simulink model "CDPR_bloques_lazo_cerrado_R2020a"  (R2020b)
settings: Solver=ode15s  StartTime=0.0  StopTime=10  MaxStep=0.001  RelTol=1e-30
InitFcn:
  | % The global parameters for simulink are defined by running this script
  | % - Back emf constant           [Kb] (V/rad/sec)
  | % - Motor torque constant       [Kt] (N.m/A)
  | % - Mechanical inertia          [Jm] (kg.m^2)
  | % - Friction coeficient         [Bm] (N.m.s)
  | % - Armature resistance         [Ra] (Ohm)
  | % - Armature inductance         [La] (H)
  | 
  | Kb = 1.25;
  | Kt = 0.516;
  | Jm = 0.0221;
  | Bm = 0.002953;
  | Ra = 2.581;
  | La = 0.0281;
  | b = 0.1;
  | m = 0.5;
  | g = 9.81;
  | r = 0.3;
settings Model: OrderedModelArguments=off  Creator=C20256  LastModifiedBy=C20256
settings DebuggingCC: AlgebraicLoopMsg=none

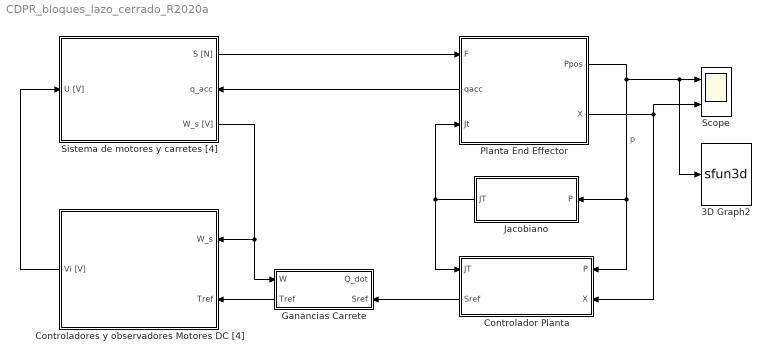
== system CDPR_bloques_lazo_cerrado_R2020a ==
  3D Graph2 : S-Function  LoadFcn=if exist('sfun3d','file'), sfun3d([],[],[],'LoadBlock'); end  FunctionName=sfun3d  Parameters=ax,T,np,cp,gd,ls,mk,mx,hd,tb  SFunctionDeploymentMode=off  EnableBusSupport=off  mask(3D Graph){np=1, ax=[-20 20 -20 20 0 20], mx=1e4, T=0.1, cp=[20 50 0.1], gd=on, hd=off, tb=off, ls=-, mk=none}
      mask prompts: np "Number of moving points (lines)"; ax "Range: [xmin xmax  ymin ymax zmin zmax]"; mx "Max number of points in each line"; T "Sampling Time"; cp "Camera position (use [0 0 1] for 2D XY view)"; gd "Grid (on|off)"; hd "HeadMarkers (on|off)"; tb "Toolbar (on|off)"; ls "LineStyle"; mk "LineMarker"
      mask help:
      | This block plots the position of several points in the XYZ space. The input contains the coordinates of all the points (x1,y1,z1,x2,y2,z2,...).
      | The number of moving points (lines), the XYZ ranges, sampling time, camera position, and grid (among other things) can be set as mask parameters.
      settings: CopyFcn=if exist('sfun3d','file'), sfun3d([],[],[],'CopyBlock'); end  DeleteFcn=if exist('sfun3d','file'), sfun3d([],[],[],'DeleteBlock'); end  NameChangeFcn=if exist('sfun3d','file'), sfun3d([],[],[],'NameChange'); end
      mask Help:
      | This block plots the position of several points in the XYZ space. The input contains the coordinates of all the points (x1,y1,z1,x2,y2,z2,...).
      | The number of moving points (lines), the XYZ ranges, sampling time, camera position, and grid (among other things) can be set as mask parameters.
      mask TypeOptions ls: - | -- | : | -. | none
      mask TypeOptions mk: none | . | + | o | * | x | square | diamond | v | ^ | > | < | pentagram | hexagram
      mask Display: plot([.05 .95 .95 .05 .05],[.45 .45 .95 .95 .45], 0.5+cos(0:0.1:2*pi)*0.3,0.7+sin(0:0.1:2*pi)*0.2)
  Controlador Planta : Subsystem
      settings: PortSchema="{\"entries\":[{\"content\":{\"sides\":[{\"content\":{\"connectorIds\":[\"In1\",\"Out1\"]},\"type\":\"ConnectorPlacement.EquallySpacedRectSide\",\"uuid\":\"e435b17b-c2fe-4911-bfed-03351310c969\"},{\"content\":{\"connectorIds\":[\"In2\",\"In3\"],\"side\":\"RIGHT\"},\"type\":\"ConnectorPlacement.EquallySpacedRectSide\",\"uuid\":\"de4daf8e-4374-4970-b69a-ffc749c87b1a\"},{\"content\":{\"connectorIds\":[],\"side\":\"TOP\"},\"type\":\"ConnectorPlacement.EquallySpacedRectSide\",\"uuid\":\"7861d55a-b03c-4daa-b9ee-ff2ad3262c5d\"}]},\"type\":\"ConnectorPlacement.EquallySpacedConnector\",\"uuid\":\"ff68927d-1fa0-407f-8d33-41a83477036e\"}],\"packageUris\":[\"http://schema.mathworks.com/mf0/Connector/19700101\"],\"version\":\"1.0\"}"
  "Controladores y observadores Motores DC [4] " : Subsystem
  Ganancias Carrete : Subsystem
      settings: PortSchema="{\"entries\":[{\"content\":{\"sides\":[{\"content\":{\"connectorIds\":[\"Out2\",\"In1\"]},\"type\":\"ConnectorPlacement.EquallySpacedRectSide\",\"uuid\":\"555f6f3e-9569-47b6-b4e7-da4822ff9d9a\"},{\"content\":{\"connectorIds\":[\"In2\",\"Out1\"],\"side\":\"RIGHT\"},\"type\":\"ConnectorPlacement.EquallySpacedRectSide\",\"uuid\":\"c772589d-41ed-413e-ad09-6c9739d0b592\"},{\"content\":{\"connectorIds\":[],\"side\":\"TOP\"},\"type\":\"ConnectorPlacement.EquallySpacedRectSide\",\"uuid\":\"476524e9-c7c1-4526-81dc-b8c364e0e521\"},{\"content\":{\"connectorIds\":[],\"side\":\"HIDDEN\"},\"type\":\"ConnectorPlacement.EquallySpacedRectSide\",\"uuid\":\"c2e2d7d4-0ad6-4cbf-86a5-e641e5a11bb7\"}]},\"type\":\"ConnectorPlacement.EquallySpacedConnector\",\"uuid\":\"74b68917-a397-45e1-97b6-aba9e759a2e3\"}],\"packageUris\":[\"http://schema.mathworks.com/mf0/Connector/R2020b\"],\"version\":\"1.0\"}"
  Jacobiano : Subsystem
  Planta End Effector : Subsystem
      settings: PortSchema="{\"entries\":[{\"content\":{\"sides\":[{\"content\":{\"connectorIds\":[\"In1\",\"Out3\",\"In2\"]},\"type\":\"ConnectorPlacement.EquallySpacedRectSide\",\"uuid\":\"e435b17b-c2fe-4911-bfed-03351310c969\"},{\"content\":{\"connectorIds\":[\"Out1\",\"Out2\"],\"side\":\"RIGHT\"},\"type\":\"ConnectorPlacement.EquallySpacedRectSide\",\"uuid\":\"de4daf8e-4374-4970-b69a-ffc749c87b1a\"},{\"content\":{\"connectorIds\":[],\"side\":\"TOP\"},\"type\":\"ConnectorPlacement.EquallySpacedRectSide\",\"uuid\":\"7861d55a-b03c-4daa-b9ee-ff2ad3262c5d\"}]},\"type\":\"ConnectorPlacement.EquallySpacedConnector\",\"uuid\":\"ff68927d-1fa0-407f-8d33-41a83477036e\"}],\"packageUris\":[\"http://schema.mathworks.com/mf0/Connector/19700101\"],\"version\":\"1.0\"}"
  Scope : Scope  NumInputPorts=2
  Sistema de motores y carretes [4] : Subsystem
      settings: PortSchema="{\"entries\":[{\"content\":{\"sides\":[{\"content\":{\"connectorIds\":[\"In1\"]},\"type\":\"ConnectorPlacement.EquallySpacedRectSide\",\"uuid\":\"f217a000-e252-4a50-bf31-1ff909748d21\"},{\"content\":{\"connectorIds\":[\"Out1\",\"In2\",\"Out2\"],\"side\":\"RIGHT\"},\"type\":\"ConnectorPlacement.EquallySpacedRectSide\",\"uuid\":\"c07a322d-5651-46c6-b0ed-f5d5b0eec680\"},{\"content\":{\"connectorIds\":[],\"side\":\"TOP\"},\"type\":\"ConnectorPlacement.EquallySpacedRectSide\",\"uuid\":\"7d447df9-94e4-4955-b02b-7a0185d62a70\"}]},\"type\":\"ConnectorPlacement.EquallySpacedConnector\",\"uuid\":\"49638b45-1ce8-4db4-875b-f1b328579de2\"}],\"packageUris\":[\"http://schema.mathworks.com/mf0/Connector/19700101\"],\"version\":\"1.0\"}"
  wires:
  Planta End Effector/1(Ppos) -> Controlador Planta/2(P), Jacobiano/1(P), 3D Graph2/1, Scope/1  "p"
  "Controladores y observadores Motores DC [4] "/1(Vi [V]) -> Sistema de motores y carretes [4]/1(U [V])
  Sistema de motores y carretes [4]/2(W_s [V]) -> Ganancias Carrete/2(W), "Controladores y observadores Motores DC [4] "/1(W_s)
  Sistema de motores y carretes [4]/1(S [N]) -> Planta End Effector/1(F)
  Planta End Effector/3(qacc) -> Sistema de motores y carretes [4]/2(q_acc)
  Jacobiano/1(JT) -> Planta End Effector/2(Jt), Controlador Planta/1(JT)
  Ganancias Carrete/1(Tref) -> "Controladores y observadores Motores DC [4] "/2(Tref)
  Controlador Planta/1(Sref) -> Ganancias Carrete/1(Sref)
  Planta End Effector/2(X) -> Controlador Planta/3(X), Scope/2

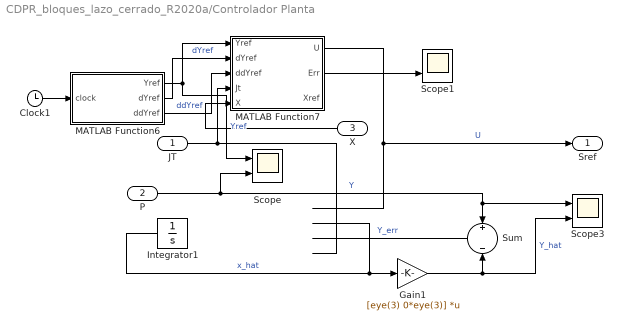
== system CDPR_bloques_lazo_cerrado_R2020a/Controlador Planta ==
  JT : Inport
  P : Inport  Port=2
  X : Inport  Port=3
  Clock1 : Clock
  Gain1 : Gain  Gain=[eye(3) 0*eye(3)]  Multiplication=Matrix(K*u)
  Integrator1 : Integrator  InitialCondition=[0 0 0 0 0 0]
  MATLAB Function6 : MATLAB Function  TreatAsAtomicUnit=on
  MATLAB Function7 : MATLAB Function  TreatAsAtomicUnit=on
  Scope : Scope  NumInputPorts=2
  Scope1 : Scope  NumInputPorts=2
  Scope3 : Scope  NumInputPorts=2
  Sum : Sum  Inputs=+||||-
  Sref : Outport
  wires:
  Integrator1/1 -> Gain1/1  "x_hat"
  ? -> Integrator1/1
  Sum/1 -> ?  "Y_err"
  Gain1/1 -> Sum/2, Scope3/2  "Y_hat"
  P/1 -> Scope/2, Scope3/1, Sum/1  "Y"
  MATLAB Function7/1(U) -> Sref/1  "U"
  MATLAB Function6/1(Yref) -> Scope/1, MATLAB Function7/1(Yref)  "Yref"
  MATLAB Function6/2(dYref) -> MATLAB Function7/2(dYref)  "dYref"
  MATLAB Function6/3(ddYref) -> MATLAB Function7/3(ddYref)  "ddYref"
  Clock1/1 -> MATLAB Function6/1(clock)
  JT/1 -> MATLAB Function7/4(Jt)
  X/1 -> MATLAB Function7/5(X)
  MATLAB Function7/2(Err) -> Scope1/2

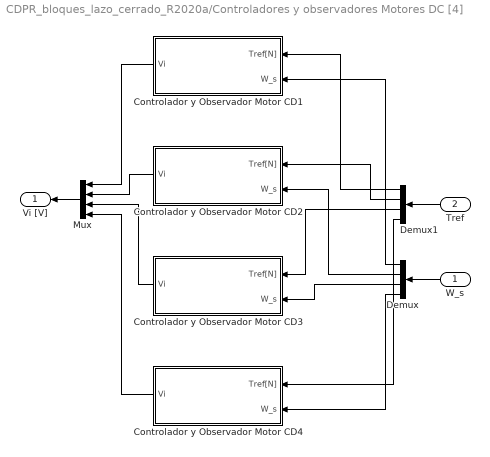
== system CDPR_bloques_lazo_cerrado_R2020a/Controladores y observadores Motores DC [4]  ==
  W_s : Inport
  Tref : Inport  Port=2
  Controlador y Observador Motor CD1 : Subsystem
      settings: PortSchema="{\"entries\":[{\"content\":{\"sides\":[{\"content\":{\"connectorIds\":[\"Out1\"]},\"type\":\"ConnectorPlacement.EquallySpacedRectSide\",\"uuid\":\"e435b17b-c2fe-4911-bfed-03351310c969\"},{\"content\":{\"connectorIds\":[\"In1\",\"In2\"],\"side\":\"RIGHT\"},\"type\":\"ConnectorPlacement.EquallySpacedRectSide\",\"uuid\":\"de4daf8e-4374-4970-b69a-ffc749c87b1a\"},{\"content\":{\"connectorIds\":[],\"side\":\"TOP\"},\"type\":\"ConnectorPlacement.EquallySpacedRectSide\",\"uuid\":\"7861d55a-b03c-4daa-b9ee-ff2ad3262c5d\"}]},\"type\":\"ConnectorPlacement.EquallySpacedConnector\",\"uuid\":\"ff68927d-1fa0-407f-8d33-41a83477036e\"}],\"packageUris\":[\"http://schema.mathworks.com/mf0/Connector/19700101\"],\"version\":\"1.0\"}"
  Controlador y Observador Motor CD2 : Subsystem
      settings: PortSchema="{\"entries\":[{\"content\":{\"sides\":[{\"content\":{\"connectorIds\":[\"Out1\"]},\"type\":\"ConnectorPlacement.EquallySpacedRectSide\",\"uuid\":\"e435b17b-c2fe-4911-bfed-03351310c969\"},{\"content\":{\"connectorIds\":[\"In1\",\"In2\"],\"side\":\"RIGHT\"},\"type\":\"ConnectorPlacement.EquallySpacedRectSide\",\"uuid\":\"de4daf8e-4374-4970-b69a-ffc749c87b1a\"},{\"content\":{\"connectorIds\":[],\"side\":\"TOP\"},\"type\":\"ConnectorPlacement.EquallySpacedRectSide\",\"uuid\":\"7861d55a-b03c-4daa-b9ee-ff2ad3262c5d\"}]},\"type\":\"ConnectorPlacement.EquallySpacedConnector\",\"uuid\":\"ff68927d-1fa0-407f-8d33-41a83477036e\"}],\"packageUris\":[\"http://schema.mathworks.com/mf0/Connector/19700101\"],\"version\":\"1.0\"}"
  Controlador y Observador Motor CD3 : Subsystem
      settings: PortSchema="{\"entries\":[{\"content\":{\"sides\":[{\"content\":{\"connectorIds\":[\"Out1\"]},\"type\":\"ConnectorPlacement.EquallySpacedRectSide\",\"uuid\":\"e435b17b-c2fe-4911-bfed-03351310c969\"},{\"content\":{\"connectorIds\":[\"In1\",\"In2\"],\"side\":\"RIGHT\"},\"type\":\"ConnectorPlacement.EquallySpacedRectSide\",\"uuid\":\"de4daf8e-4374-4970-b69a-ffc749c87b1a\"},{\"content\":{\"connectorIds\":[],\"side\":\"TOP\"},\"type\":\"ConnectorPlacement.EquallySpacedRectSide\",\"uuid\":\"7861d55a-b03c-4daa-b9ee-ff2ad3262c5d\"}]},\"type\":\"ConnectorPlacement.EquallySpacedConnector\",\"uuid\":\"ff68927d-1fa0-407f-8d33-41a83477036e\"}],\"packageUris\":[\"http://schema.mathworks.com/mf0/Connector/19700101\"],\"version\":\"1.0\"}"
  Controlador y Observador Motor CD4 : Subsystem
      settings: PortSchema="{\"entries\":[{\"content\":{\"sides\":[{\"content\":{\"connectorIds\":[\"Out1\"]},\"type\":\"ConnectorPlacement.EquallySpacedRectSide\",\"uuid\":\"e435b17b-c2fe-4911-bfed-03351310c969\"},{\"content\":{\"connectorIds\":[\"In1\",\"In2\"],\"side\":\"RIGHT\"},\"type\":\"ConnectorPlacement.EquallySpacedRectSide\",\"uuid\":\"de4daf8e-4374-4970-b69a-ffc749c87b1a\"},{\"content\":{\"connectorIds\":[],\"side\":\"TOP\"},\"type\":\"ConnectorPlacement.EquallySpacedRectSide\",\"uuid\":\"7861d55a-b03c-4daa-b9ee-ff2ad3262c5d\"}]},\"type\":\"ConnectorPlacement.EquallySpacedConnector\",\"uuid\":\"ff68927d-1fa0-407f-8d33-41a83477036e\"}],\"packageUris\":[\"http://schema.mathworks.com/mf0/Connector/19700101\"],\"version\":\"1.0\"}"
  Demux : Demux
  Demux1 : Demux
  Mux : Mux
  Vi [V] : Outport
  wires:
  W_s/1 -> Demux/1
  Tref/1 -> Demux1/1
  Demux1/1 -> Controlador y Observador Motor CD1/1(Tref[N])
  Demux1/2 -> Controlador y Observador Motor CD2/1(Tref[N])
  Demux1/3 -> Controlador y Observador Motor CD3/1(Tref[N])
  Demux1/4 -> Controlador y Observador Motor CD4/1(Tref[N])
  Demux/1 -> Controlador y Observador Motor CD1/2(W_s)
  Demux/2 -> Controlador y Observador Motor CD2/2(W_s)
  Demux/3 -> Controlador y Observador Motor CD3/2(W_s)
  Demux/4 -> Controlador y Observador Motor CD4/2(W_s)
  Controlador y Observador Motor CD4/1(Vi) -> Mux/4
  Controlador y Observador Motor CD3/1(Vi) -> Mux/3
  Mux/1 -> Vi [V]/1
  Controlador y Observador Motor CD2/1(Vi) -> Mux/2
  Controlador y Observador Motor CD1/1(Vi) -> Mux/1

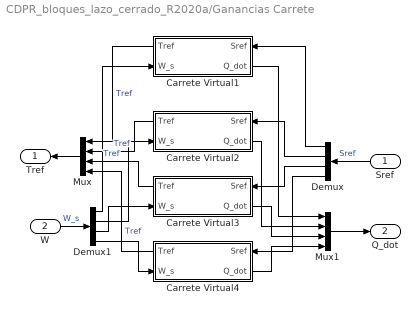
== system CDPR_bloques_lazo_cerrado_R2020a/Ganancias Carrete ==
  Sref : Inport
  W : Inport  Port=2
  Carrete Virtual1 : Subsystem
      settings: PortSchema="{\"entries\":[{\"content\":{\"sides\":[{\"content\":{\"connectorIds\":[\"In1\",\"Out2\"]},\"type\":\"ConnectorPlacement.EquallySpacedRectSide\",\"uuid\":\"555f6f3e-9569-47b6-b4e7-da4822ff9d9a\"},{\"content\":{\"connectorIds\":[\"Out1\",\"In2\"],\"side\":\"RIGHT\"},\"type\":\"ConnectorPlacement.EquallySpacedRectSide\",\"uuid\":\"c772589d-41ed-413e-ad09-6c9739d0b592\"},{\"content\":{\"connectorIds\":[],\"side\":\"TOP\"},\"type\":\"ConnectorPlacement.EquallySpacedRectSide\",\"uuid\":\"476524e9-c7c1-4526-81dc-b8c364e0e521\"},{\"content\":{\"connectorIds\":[],\"side\":\"HIDDEN\"},\"type\":\"ConnectorPlacement.EquallySpacedRectSide\",\"uuid\":\"c2e2d7d4-0ad6-4cbf-86a5-e641e5a11bb7\"}]},\"type\":\"ConnectorPlacement.EquallySpacedConnector\",\"uuid\":\"74b68917-a397-45e1-97b6-aba9e759a2e3\"}],\"packageUris\":[\"http://schema.mathworks.com/mf0/Connector/R2020b\"],\"version\":\"1.0\"}"
  Carrete Virtual2 : Subsystem
      settings: PortSchema="{\"entries\":[{\"content\":{\"sides\":[{\"content\":{\"connectorIds\":[\"In1\",\"Out2\"]},\"type\":\"ConnectorPlacement.EquallySpacedRectSide\",\"uuid\":\"555f6f3e-9569-47b6-b4e7-da4822ff9d9a\"},{\"content\":{\"connectorIds\":[\"Out1\",\"In2\"],\"side\":\"RIGHT\"},\"type\":\"ConnectorPlacement.EquallySpacedRectSide\",\"uuid\":\"c772589d-41ed-413e-ad09-6c9739d0b592\"},{\"content\":{\"connectorIds\":[],\"side\":\"TOP\"},\"type\":\"ConnectorPlacement.EquallySpacedRectSide\",\"uuid\":\"476524e9-c7c1-4526-81dc-b8c364e0e521\"},{\"content\":{\"connectorIds\":[],\"side\":\"HIDDEN\"},\"type\":\"ConnectorPlacement.EquallySpacedRectSide\",\"uuid\":\"c2e2d7d4-0ad6-4cbf-86a5-e641e5a11bb7\"}]},\"type\":\"ConnectorPlacement.EquallySpacedConnector\",\"uuid\":\"74b68917-a397-45e1-97b6-aba9e759a2e3\"}],\"packageUris\":[\"http://schema.mathworks.com/mf0/Connector/R2020b\"],\"version\":\"1.0\"}"
  Carrete Virtual3 : Subsystem
      settings: PortSchema="{\"entries\":[{\"content\":{\"sides\":[{\"content\":{\"connectorIds\":[\"In1\",\"Out2\"]},\"type\":\"ConnectorPlacement.EquallySpacedRectSide\",\"uuid\":\"555f6f3e-9569-47b6-b4e7-da4822ff9d9a\"},{\"content\":{\"connectorIds\":[\"Out1\",\"In2\"],\"side\":\"RIGHT\"},\"type\":\"ConnectorPlacement.EquallySpacedRectSide\",\"uuid\":\"c772589d-41ed-413e-ad09-6c9739d0b592\"},{\"content\":{\"connectorIds\":[],\"side\":\"TOP\"},\"type\":\"ConnectorPlacement.EquallySpacedRectSide\",\"uuid\":\"476524e9-c7c1-4526-81dc-b8c364e0e521\"},{\"content\":{\"connectorIds\":[],\"side\":\"HIDDEN\"},\"type\":\"ConnectorPlacement.EquallySpacedRectSide\",\"uuid\":\"c2e2d7d4-0ad6-4cbf-86a5-e641e5a11bb7\"}]},\"type\":\"ConnectorPlacement.EquallySpacedConnector\",\"uuid\":\"74b68917-a397-45e1-97b6-aba9e759a2e3\"}],\"packageUris\":[\"http://schema.mathworks.com/mf0/Connector/R2020b\"],\"version\":\"1.0\"}"
  Carrete Virtual4 : Subsystem
      settings: PortSchema="{\"entries\":[{\"content\":{\"sides\":[{\"content\":{\"connectorIds\":[\"In1\",\"Out2\"]},\"type\":\"ConnectorPlacement.EquallySpacedRectSide\",\"uuid\":\"555f6f3e-9569-47b6-b4e7-da4822ff9d9a\"},{\"content\":{\"connectorIds\":[\"Out1\",\"In2\"],\"side\":\"RIGHT\"},\"type\":\"ConnectorPlacement.EquallySpacedRectSide\",\"uuid\":\"c772589d-41ed-413e-ad09-6c9739d0b592\"},{\"content\":{\"connectorIds\":[],\"side\":\"TOP\"},\"type\":\"ConnectorPlacement.EquallySpacedRectSide\",\"uuid\":\"476524e9-c7c1-4526-81dc-b8c364e0e521\"},{\"content\":{\"connectorIds\":[],\"side\":\"HIDDEN\"},\"type\":\"ConnectorPlacement.EquallySpacedRectSide\",\"uuid\":\"c2e2d7d4-0ad6-4cbf-86a5-e641e5a11bb7\"}]},\"type\":\"ConnectorPlacement.EquallySpacedConnector\",\"uuid\":\"74b68917-a397-45e1-97b6-aba9e759a2e3\"}],\"packageUris\":[\"http://schema.mathworks.com/mf0/Connector/R2020b\"],\"version\":\"1.0\"}"
  Demux : Demux
  Demux1 : Demux
  Mux : Mux
  Mux1 : Mux
  Tref : Outport
  Q_dot : Outport  Port=2
  wires:
  Sref/1 -> Demux/1  "Sref"
  Demux/1 -> Carrete Virtual1/1(Sref)
  Carrete Virtual1/1(Tref) -> Mux/1  "Tref"
  Demux/2 -> Carrete Virtual2/1(Sref)
  Demux/3 -> Carrete Virtual3/1(Sref)
  Demux/4 -> Carrete Virtual4/1(Sref)
  Carrete Virtual2/1(Tref) -> Mux/2  "Tref"
  Carrete Virtual3/1(Tref) -> Mux/3  "Tref"
  Carrete Virtual4/1(Tref) -> Mux/4  "Tref"
  Mux/1 -> Tref/1
  W/1 -> Demux1/1  "W_s"
  Demux1/1 -> Carrete Virtual1/2(W_s)
  Demux1/2 -> Carrete Virtual2/2(W_s)
  Demux1/3 -> Carrete Virtual3/2(W_s)
  Demux1/4 -> Carrete Virtual4/2(W_s)
  Mux1/1 -> Q_dot/1
  Carrete Virtual4/2(Q_dot) -> Mux1/4
  Carrete Virtual3/2(Q_dot) -> Mux1/3
  Carrete Virtual2/2(Q_dot) -> Mux1/2
  Carrete Virtual1/2(Q_dot) -> Mux1/1

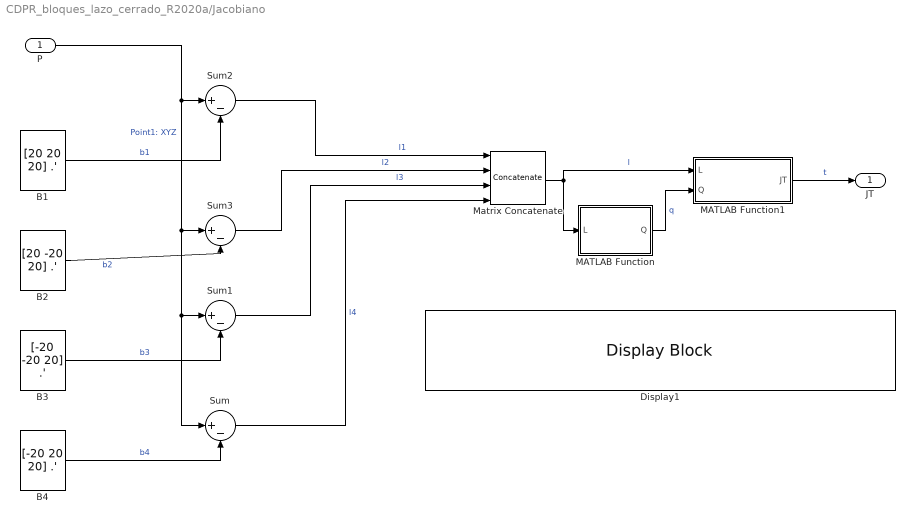
== system CDPR_bloques_lazo_cerrado_R2020a/Jacobiano ==
  P : Inport
  B1 : Constant  Value=[20 20 20] .'  VectorParams1D=off
  B2 : Constant  Value=[20 -20 20] .'  VectorParams1D=off
  B3 : Constant  Value=[-20 -20 20] .'  VectorParams1D=off
  B4 : Constant  Value=[-20 20 20] .'  VectorParams1D=off
  Display1 : DisplayBlock  LabelPosition=Hide  Format=short  Transparency=1
  MATLAB Function : MATLAB Function  TreatAsAtomicUnit=on
  MATLAB Function1 : MATLAB Function  TreatAsAtomicUnit=on
  Matrix Concatenate : Concatenate  NumInputs=4  Mode=Multidimensional array  ConcatenateDimension=2
  Sum{,1..3} (4 alike) : Sum  Inputs=|+-
  JT : Outport
  wires:
  B2/1 -> Sum3/2  "b2"
  MATLAB Function/1(Q) -> MATLAB Function1/2(Q)  "q"
  B3/1 -> Sum1/2  "b3"
  Sum/1 -> Matrix Concatenate/4  "l4"
  Matrix Concatenate/1 -> MATLAB Function1/1(L), MATLAB Function/1(L)  "l"
  Sum3/1 -> Matrix Concatenate/2  "l2"
  Sum2/1 -> Matrix Concatenate/1  "l1"
  B4/1 -> Sum/2  "b4"
  Sum1/1 -> Matrix Concatenate/3  "l3"
  B1/1 -> Sum2/2  "b1"
  P/1 -> Sum1/1, Sum/1, Sum3/1, Sum2/1  "Point1: XYZ"
  MATLAB Function1/1(JT) -> JT/1  "t"

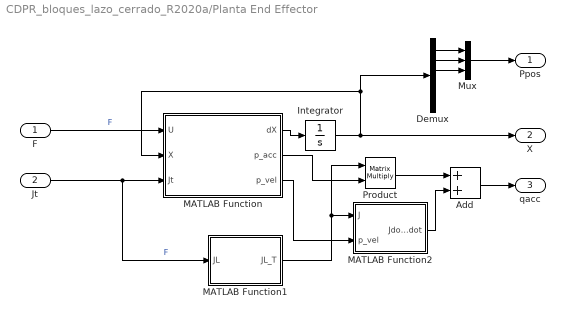
== system CDPR_bloques_lazo_cerrado_R2020a/Planta End Effector ==
  F : Inport
  Jt : Inport  Port=2
  Add : Sum
  Demux : Demux  Outputs=6
  Integrator : Integrator  InitialCondition=[0 0 0 0 0 0]
  MATLAB Function : MATLAB Function  TreatAsAtomicUnit=on
  MATLAB Function1 : MATLAB Function  TreatAsAtomicUnit=on
  MATLAB Function2 : MATLAB Function  TreatAsAtomicUnit=on
  Mux : Mux  Inputs=3
  Product : Product  Multiplication=Matrix(*)
  Ppos : Outport
  X : Outport  Port=2
  qacc : Outport  Port=3
  wires:
  Integrator/1 -> X/1, MATLAB Function/2(X), Demux/1
  MATLAB Function/1(dX) -> Integrator/1
  Mux/1 -> Ppos/1
  F/1 -> MATLAB Function/1(U)  "F"
  Jt/1 -> MATLAB Function1/1(JL), MATLAB Function/3(Jt)  "F"
  MATLAB Function/2(p_acc) -> Product/2
  MATLAB Function1/1(JL_T) -> Product/1, MATLAB Function2/1(J)
  Demux/1 -> Mux/1
  Demux/2 -> Mux/2
  Demux/3 -> Mux/3
  MATLAB Function/3(p_vel) -> MATLAB Function2/2(p_vel)
  Add/1 -> qacc/1
  Product/1 -> Add/1
  MATLAB Function2/1(JdotQdot) -> Add/2

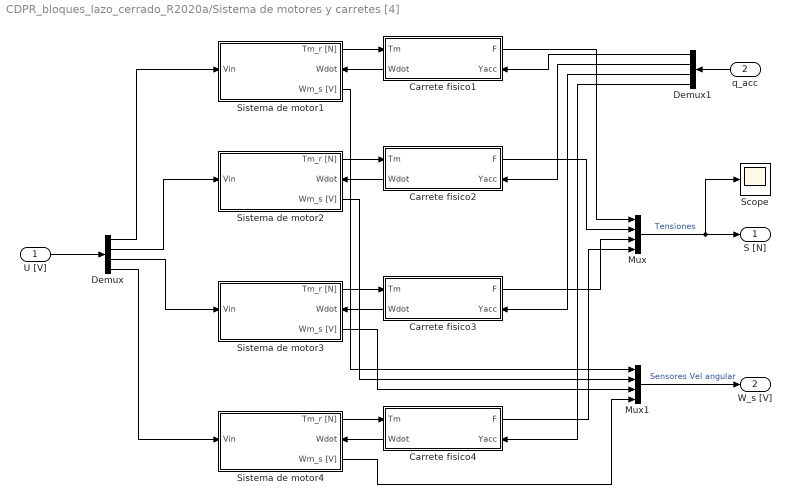
== system CDPR_bloques_lazo_cerrado_R2020a/Sistema de motores y carretes [4] ==
  U [V] : Inport
  q_acc : Inport  Port=2
  Carrete fisico1 : Subsystem
      settings: PortSchema="{\"entries\":[{\"content\":{\"sides\":[{\"content\":{\"connectorIds\":[\"In1\",\"Out2\"]},\"type\":\"ConnectorPlacement.EquallySpacedRectSide\",\"uuid\":\"e435b17b-c2fe-4911-bfed-03351310c969\"},{\"content\":{\"connectorIds\":[\"Out1\",\"In2\"],\"side\":\"RIGHT\"},\"type\":\"ConnectorPlacement.EquallySpacedRectSide\",\"uuid\":\"de4daf8e-4374-4970-b69a-ffc749c87b1a\"},{\"content\":{\"connectorIds\":[],\"side\":\"TOP\"},\"type\":\"ConnectorPlacement.EquallySpacedRectSide\",\"uuid\":\"7861d55a-b03c-4daa-b9ee-ff2ad3262c5d\"}]},\"type\":\"ConnectorPlacement.EquallySpacedConnector\",\"uuid\":\"ff68927d-1fa0-407f-8d33-41a83477036e\"}],\"packageUris\":[\"http://schema.mathworks.com/mf0/Connector/19700101\"],\"version\":\"1.0\"}"
  Carrete fisico2 : Subsystem
      settings: PortSchema="{\"entries\":[{\"content\":{\"sides\":[{\"content\":{\"connectorIds\":[\"In1\",\"Out2\"]},\"type\":\"ConnectorPlacement.EquallySpacedRectSide\",\"uuid\":\"e435b17b-c2fe-4911-bfed-03351310c969\"},{\"content\":{\"connectorIds\":[\"Out1\",\"In2\"],\"side\":\"RIGHT\"},\"type\":\"ConnectorPlacement.EquallySpacedRectSide\",\"uuid\":\"de4daf8e-4374-4970-b69a-ffc749c87b1a\"},{\"content\":{\"connectorIds\":[],\"side\":\"TOP\"},\"type\":\"ConnectorPlacement.EquallySpacedRectSide\",\"uuid\":\"7861d55a-b03c-4daa-b9ee-ff2ad3262c5d\"}]},\"type\":\"ConnectorPlacement.EquallySpacedConnector\",\"uuid\":\"ff68927d-1fa0-407f-8d33-41a83477036e\"}],\"packageUris\":[\"http://schema.mathworks.com/mf0/Connector/19700101\"],\"version\":\"1.0\"}"
  Carrete fisico3 : Subsystem
      settings: PortSchema="{\"entries\":[{\"content\":{\"sides\":[{\"content\":{\"connectorIds\":[\"In1\",\"Out2\"]},\"type\":\"ConnectorPlacement.EquallySpacedRectSide\",\"uuid\":\"e435b17b-c2fe-4911-bfed-03351310c969\"},{\"content\":{\"connectorIds\":[\"Out1\",\"In2\"],\"side\":\"RIGHT\"},\"type\":\"ConnectorPlacement.EquallySpacedRectSide\",\"uuid\":\"de4daf8e-4374-4970-b69a-ffc749c87b1a\"},{\"content\":{\"connectorIds\":[],\"side\":\"TOP\"},\"type\":\"ConnectorPlacement.EquallySpacedRectSide\",\"uuid\":\"7861d55a-b03c-4daa-b9ee-ff2ad3262c5d\"}]},\"type\":\"ConnectorPlacement.EquallySpacedConnector\",\"uuid\":\"ff68927d-1fa0-407f-8d33-41a83477036e\"}],\"packageUris\":[\"http://schema.mathworks.com/mf0/Connector/19700101\"],\"version\":\"1.0\"}"
  Carrete fisico4 : Subsystem
      settings: PortSchema="{\"entries\":[{\"content\":{\"sides\":[{\"content\":{\"connectorIds\":[\"In1\",\"Out2\"]},\"type\":\"ConnectorPlacement.EquallySpacedRectSide\",\"uuid\":\"e435b17b-c2fe-4911-bfed-03351310c969\"},{\"content\":{\"connectorIds\":[\"Out1\",\"In2\"],\"side\":\"RIGHT\"},\"type\":\"ConnectorPlacement.EquallySpacedRectSide\",\"uuid\":\"de4daf8e-4374-4970-b69a-ffc749c87b1a\"},{\"content\":{\"connectorIds\":[],\"side\":\"TOP\"},\"type\":\"ConnectorPlacement.EquallySpacedRectSide\",\"uuid\":\"7861d55a-b03c-4daa-b9ee-ff2ad3262c5d\"}]},\"type\":\"ConnectorPlacement.EquallySpacedConnector\",\"uuid\":\"ff68927d-1fa0-407f-8d33-41a83477036e\"}],\"packageUris\":[\"http://schema.mathworks.com/mf0/Connector/19700101\"],\"version\":\"1.0\"}"
  Demux : Demux
  Demux1 : Demux
  Mux : Mux
  Mux1 : Mux
  Scope : Scope
  Sistema de motor1 : Subsystem
      settings: PortSchema="{\"entries\":[{\"content\":{\"sides\":[{\"content\":{\"connectorIds\":[\"In1\"]},\"type\":\"ConnectorPlacement.EquallySpacedRectSide\",\"uuid\":\"e435b17b-c2fe-4911-bfed-03351310c969\"},{\"content\":{\"connectorIds\":[\"Out1\",\"In2\",\"Out2\"],\"side\":\"RIGHT\"},\"type\":\"ConnectorPlacement.EquallySpacedRectSide\",\"uuid\":\"de4daf8e-4374-4970-b69a-ffc749c87b1a\"},{\"content\":{\"connectorIds\":[],\"side\":\"TOP\"},\"type\":\"ConnectorPlacement.EquallySpacedRectSide\",\"uuid\":\"7861d55a-b03c-4daa-b9ee-ff2ad3262c5d\"}]},\"type\":\"ConnectorPlacement.EquallySpacedConnector\",\"uuid\":\"ff68927d-1fa0-407f-8d33-41a83477036e\"}],\"packageUris\":[\"http://schema.mathworks.com/mf0/Connector/19700101\"],\"version\":\"1.0\"}"
  Sistema de motor2 : Subsystem
      settings: PortSchema="{\"entries\":[{\"content\":{\"sides\":[{\"content\":{\"connectorIds\":[\"In1\"]},\"type\":\"ConnectorPlacement.EquallySpacedRectSide\",\"uuid\":\"e435b17b-c2fe-4911-bfed-03351310c969\"},{\"content\":{\"connectorIds\":[\"Out1\",\"In2\",\"Out2\"],\"side\":\"RIGHT\"},\"type\":\"ConnectorPlacement.EquallySpacedRectSide\",\"uuid\":\"de4daf8e-4374-4970-b69a-ffc749c87b1a\"},{\"content\":{\"connectorIds\":[],\"side\":\"TOP\"},\"type\":\"ConnectorPlacement.EquallySpacedRectSide\",\"uuid\":\"7861d55a-b03c-4daa-b9ee-ff2ad3262c5d\"}]},\"type\":\"ConnectorPlacement.EquallySpacedConnector\",\"uuid\":\"ff68927d-1fa0-407f-8d33-41a83477036e\"}],\"packageUris\":[\"http://schema.mathworks.com/mf0/Connector/19700101\"],\"version\":\"1.0\"}"
  Sistema de motor3 : Subsystem
      settings: PortSchema="{\"entries\":[{\"content\":{\"sides\":[{\"content\":{\"connectorIds\":[\"In1\"]},\"type\":\"ConnectorPlacement.EquallySpacedRectSide\",\"uuid\":\"e435b17b-c2fe-4911-bfed-03351310c969\"},{\"content\":{\"connectorIds\":[\"Out1\",\"In2\",\"Out2\"],\"side\":\"RIGHT\"},\"type\":\"ConnectorPlacement.EquallySpacedRectSide\",\"uuid\":\"de4daf8e-4374-4970-b69a-ffc749c87b1a\"},{\"content\":{\"connectorIds\":[],\"side\":\"TOP\"},\"type\":\"ConnectorPlacement.EquallySpacedRectSide\",\"uuid\":\"7861d55a-b03c-4daa-b9ee-ff2ad3262c5d\"}]},\"type\":\"ConnectorPlacement.EquallySpacedConnector\",\"uuid\":\"ff68927d-1fa0-407f-8d33-41a83477036e\"}],\"packageUris\":[\"http://schema.mathworks.com/mf0/Connector/19700101\"],\"version\":\"1.0\"}"
  Sistema de motor4 : Subsystem
      settings: PortSchema="{\"entries\":[{\"content\":{\"sides\":[{\"content\":{\"connectorIds\":[\"In1\"]},\"type\":\"ConnectorPlacement.EquallySpacedRectSide\",\"uuid\":\"e435b17b-c2fe-4911-bfed-03351310c969\"},{\"content\":{\"connectorIds\":[\"Out1\",\"In2\",\"Out2\"],\"side\":\"RIGHT\"},\"type\":\"ConnectorPlacement.EquallySpacedRectSide\",\"uuid\":\"de4daf8e-4374-4970-b69a-ffc749c87b1a\"},{\"content\":{\"connectorIds\":[],\"side\":\"TOP\"},\"type\":\"ConnectorPlacement.EquallySpacedRectSide\",\"uuid\":\"7861d55a-b03c-4daa-b9ee-ff2ad3262c5d\"}]},\"type\":\"ConnectorPlacement.EquallySpacedConnector\",\"uuid\":\"ff68927d-1fa0-407f-8d33-41a83477036e\"}],\"packageUris\":[\"http://schema.mathworks.com/mf0/Connector/19700101\"],\"version\":\"1.0\"}"
  S [N] : Outport
  W_s [V] : Outport  Port=2
  wires:
  Sistema de motor3/2(Wm_s [V]) -> Mux1/3
  Carrete fisico3/2(Wdot) -> Sistema de motor3/2(Wdot)
  Sistema de motor1/2(Wm_s [V]) -> Mux1/1
  Carrete fisico2/2(Wdot) -> Sistema de motor2/2(Wdot)
  Sistema de motor3/1(Tm_r [N]) -> Carrete fisico3/1(Tm)
  Sistema de motor4/2(Wm_s [V]) -> Mux1/4
  Sistema de motor1/1(Tm_r [N]) -> Carrete fisico1/1(Tm)
  Sistema de motor2/2(Wm_s [V]) -> Mux1/2
  Carrete fisico4/2(Wdot) -> Sistema de motor4/2(Wdot)
  Sistema de motor2/1(Tm_r [N]) -> Carrete fisico2/1(Tm)
  Carrete fisico1/2(Wdot) -> Sistema de motor1/2(Wdot)
  Sistema de motor4/1(Tm_r [N]) -> Carrete fisico4/1(Tm)
  Demux/1 -> Sistema de motor1/1(Vin)
  Demux/2 -> Sistema de motor2/1(Vin)
  Demux/3 -> Sistema de motor3/1(Vin)
  Demux/4 -> Sistema de motor4/1(Vin)
  U [V]/1 -> Demux/1
  Carrete fisico2/1(F) -> Mux/2
  Carrete fisico1/1(F) -> Mux/1
  Carrete fisico3/1(F) -> Mux/3
  Carrete fisico4/1(F) -> Mux/4
  Mux1/1 -> W_s [V]/1  "Sensores Vel angular"
  Mux/1 -> Scope/1, S [N]/1  "Tensiones"
  q_acc/1 -> Demux1/1
  Demux1/1 -> Carrete fisico1/2(Yacc)
  Demux1/2 -> Carrete fisico2/2(Yacc)
  Demux1/3 -> Carrete fisico3/2(Yacc)
  Demux1/4 -> Carrete fisico4/2(Yacc)

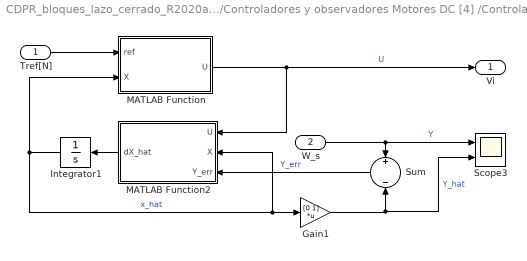
== system CDPR_bloques_lazo_cerrado_R2020a/Controladores y observadores Motores DC [4] /Controlador y Observador Motor CD1 ==
  Tref[N] : Inport
  W_s : Inport  Port=2
  Gain1 : Gain  Gain=[0 1]  Multiplication=Matrix(K*u)
  Integrator1 : Integrator  InitialCondition=[0 0]
  MATLAB Function : MATLAB Function  TreatAsAtomicUnit=on
  MATLAB Function2 : MATLAB Function  TreatAsAtomicUnit=on
  Scope3 : Scope  NumInputPorts=2
  Sum : Sum  Inputs=+||||-
  Vi : Outport
  wires:
  Integrator1/1 -> MATLAB Function/2(X), Gain1/1, MATLAB Function2/2(X)  "x_hat"
  MATLAB Function2/1(dX_hat) -> Integrator1/1
  Sum/1 -> MATLAB Function2/3(Y_err)  "Y_err"
  Tref[N]/1 -> MATLAB Function/1(ref)
  Gain1/1 -> Scope3/2, Sum/2  "Y_hat"
  W_s/1 -> Scope3/1, Sum/1  "Y"
  MATLAB Function/1(U) -> Vi/1, MATLAB Function2/1(U)  "U"

== system CDPR_bloques_lazo_cerrado_R2020a/Controladores y observadores Motores DC [4] /Controlador y Observador Motor CD2 ==
  Tref[N] : Inport
  W_s : Inport  Port=2
  Gain1 : Gain  Gain=[0 1]  Multiplication=Matrix(K*u)
  Integrator1 : Integrator  InitialCondition=[0 0]
  MATLAB Function : MATLAB Function  TreatAsAtomicUnit=on
  MATLAB Function2 : MATLAB Function  TreatAsAtomicUnit=on
  Scope3 : Scope  NumInputPorts=2
  Sum : Sum  Inputs=+||||-
  Vi : Outport
  wires:
  Integrator1/1 -> MATLAB Function/2(X), Gain1/1, MATLAB Function2/2(X)  "x_hat"
  MATLAB Function2/1(dX_hat) -> Integrator1/1
  Sum/1 -> MATLAB Function2/3(Y_err)  "Y_err"
  Tref[N]/1 -> MATLAB Function/1(ref)
  Gain1/1 -> Scope3/2, Sum/2  "Y_hat"
  W_s/1 -> Scope3/1, Sum/1  "Y"
  MATLAB Function/1(U) -> Vi/1, MATLAB Function2/1(U)  "U"

== system CDPR_bloques_lazo_cerrado_R2020a/Controladores y observadores Motores DC [4] /Controlador y Observador Motor CD3 ==
  Tref[N] : Inport
  W_s : Inport  Port=2
  Gain1 : Gain  Gain=[0 1]  Multiplication=Matrix(K*u)
  Integrator1 : Integrator  InitialCondition=[0 0]
  MATLAB Function : MATLAB Function  TreatAsAtomicUnit=on
  MATLAB Function2 : MATLAB Function  TreatAsAtomicUnit=on
  Scope3 : Scope  NumInputPorts=2
  Sum : Sum  Inputs=+||||-
  Vi : Outport
  wires:
  Integrator1/1 -> MATLAB Function/2(X), Gain1/1, MATLAB Function2/2(X)  "x_hat"
  MATLAB Function2/1(dX_hat) -> Integrator1/1
  Sum/1 -> MATLAB Function2/3(Y_err)  "Y_err"
  Tref[N]/1 -> MATLAB Function/1(ref)
  Gain1/1 -> Scope3/2, Sum/2  "Y_hat"
  W_s/1 -> Scope3/1, Sum/1  "Y"
  MATLAB Function/1(U) -> Vi/1, MATLAB Function2/1(U)  "U"

== system CDPR_bloques_lazo_cerrado_R2020a/Controladores y observadores Motores DC [4] /Controlador y Observador Motor CD4 ==
  Tref[N] : Inport
  W_s : Inport  Port=2
  Gain1 : Gain  Gain=[0 1]  Multiplication=Matrix(K*u)
  Integrator1 : Integrator  InitialCondition=[0 0]
  MATLAB Function : MATLAB Function  TreatAsAtomicUnit=on
  MATLAB Function2 : MATLAB Function  TreatAsAtomicUnit=on
  Scope3 : Scope  NumInputPorts=2
  Sum : Sum  Inputs=+||||-
  Vi : Outport
  wires:
  Integrator1/1 -> MATLAB Function/2(X), Gain1/1, MATLAB Function2/2(X)  "x_hat"
  MATLAB Function2/1(dX_hat) -> Integrator1/1
  Sum/1 -> MATLAB Function2/3(Y_err)  "Y_err"
  Tref[N]/1 -> MATLAB Function/1(ref)
  Gain1/1 -> Scope3/2, Sum/2  "Y_hat"
  W_s/1 -> Scope3/1, Sum/1  "Y"
  MATLAB Function/1(U) -> Vi/1, MATLAB Function2/1(U)  "U"

== system CDPR_bloques_lazo_cerrado_R2020a/Ganancias Carrete/Carrete Virtual1 ==
  Sref : Inport
  W_s : Inport  Port=2
  Gain : Gain  Gain=0.005
  Gain1 : Gain  Gain=0.005
  Tref : Outport
  Q_dot : Outport  Port=2
  wires:
  Sref/1 -> Gain/1  "Sref"
  Gain/1 -> Tref/1  "Tref"
  Gain1/1 -> Q_dot/1  "Vel Lin"
  W_s/1 -> Gain1/1  "Vel ang"

== system CDPR_bloques_lazo_cerrado_R2020a/Ganancias Carrete/Carrete Virtual2 ==
  Sref : Inport
  W_s : Inport  Port=2
  Gain : Gain  Gain=0.005
  Gain1 : Gain  Gain=0.005
  Tref : Outport
  Q_dot : Outport  Port=2
  wires:
  Sref/1 -> Gain/1  "Sref"
  Gain/1 -> Tref/1  "Tref"
  Gain1/1 -> Q_dot/1  "Vel Lin"
  W_s/1 -> Gain1/1  "Vel ang"

== system CDPR_bloques_lazo_cerrado_R2020a/Ganancias Carrete/Carrete Virtual3 ==
  Sref : Inport
  W_s : Inport  Port=2
  Gain : Gain  Gain=0.005
  Gain1 : Gain  Gain=0.005
  Tref : Outport
  Q_dot : Outport  Port=2
  wires:
  Sref/1 -> Gain/1  "Sref"
  Gain/1 -> Tref/1  "Tref"
  Gain1/1 -> Q_dot/1  "Vel Lin"
  W_s/1 -> Gain1/1  "Vel ang"

== system CDPR_bloques_lazo_cerrado_R2020a/Ganancias Carrete/Carrete Virtual4 ==
  Sref : Inport
  W_s : Inport  Port=2
  Gain : Gain  Gain=0.005
  Gain1 : Gain  Gain=0.005
  Tref : Outport
  Q_dot : Outport  Port=2
  wires:
  Sref/1 -> Gain/1  "Sref"
  Gain/1 -> Tref/1  "Tref"
  Gain1/1 -> Q_dot/1  "Vel Lin"
  W_s/1 -> Gain1/1  "Vel ang"

== system CDPR_bloques_lazo_cerrado_R2020a/Sistema de motores y carretes [4]/Carrete fisico1 ==
  Tm : Inport
  Yacc : Inport  Port=2
  Gain : Gain  Gain=1/0.005
  Gain1 : Gain  Gain=1/0.005
  F : Outport
  Wdot : Outport  Port=2
  wires:
  Tm/1 -> Gain/1  "Tm"
  Gain/1 -> F/1  "F"
  Yacc/1 -> Gain1/1  "Yacc"
  Gain1/1 -> Wdot/1  "Acc ang"

== system CDPR_bloques_lazo_cerrado_R2020a/Sistema de motores y carretes [4]/Carrete fisico2 ==
  Tm : Inport
  Yacc : Inport  Port=2
  Gain : Gain  Gain=1/0.005
  Gain1 : Gain  Gain=1/0.005
  F : Outport
  Wdot : Outport  Port=2
  wires:
  Tm/1 -> Gain/1  "Tm"
  Gain/1 -> F/1  "F"
  Yacc/1 -> Gain1/1  "Yacc"
  Gain1/1 -> Wdot/1  "Acc ang"

== system CDPR_bloques_lazo_cerrado_R2020a/Sistema de motores y carretes [4]/Carrete fisico3 ==
  Tm : Inport
  Yacc : Inport  Port=2
  Gain : Gain  Gain=1/0.005
  Gain1 : Gain  Gain=1/0.005
  F : Outport
  Wdot : Outport  Port=2
  wires:
  Tm/1 -> Gain/1  "Tm"
  Gain/1 -> F/1  "F"
  Yacc/1 -> Gain1/1  "Yacc"
  Gain1/1 -> Wdot/1  "Acc ang"

== system CDPR_bloques_lazo_cerrado_R2020a/Sistema de motores y carretes [4]/Carrete fisico4 ==
  Tm : Inport
  Yacc : Inport  Port=2
  Gain : Gain  Gain=1/0.005
  Gain1 : Gain  Gain=1/0.005
  F : Outport
  Wdot : Outport  Port=2
  wires:
  Tm/1 -> Gain/1  "Tm"
  Gain/1 -> F/1  "F"
  Yacc/1 -> Gain1/1  "Yacc"
  Gain1/1 -> Wdot/1  "Acc ang"

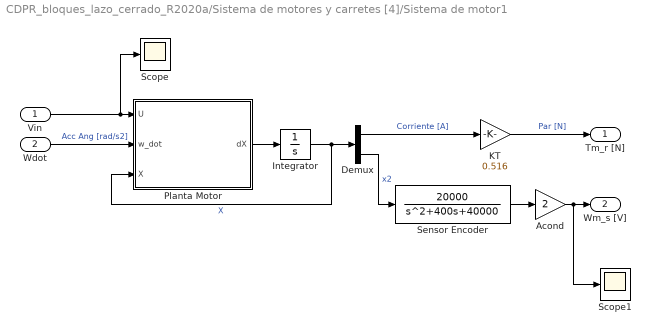
== system CDPR_bloques_lazo_cerrado_R2020a/Sistema de motores y carretes [4]/Sistema de motor1 ==
  Vin : Inport
  Wdot : Inport  Port=2
  Acond : Gain  Gain=2
  Demux : Demux  Outputs=2
  Integrator : Integrator  InitialCondition=[0 0]
  KT : Gain  Gain=0.516
  Planta Motor : MATLAB Function  TreatAsAtomicUnit=on
  Scope : Scope
  Scope1 : Scope
  Sensor Encoder : TransferFcn  Numerator=[20000]  Denominator=[1 400 40000]
  Tm_r [N] : Outport
  Wm_s [V] : Outport  Port=2
  wires:
  Planta Motor/1(dX) -> Integrator/1
  Integrator/1 -> Planta Motor/3(X), Demux/1  "X"
  KT/1 -> Tm_r [N]/1  "Par [N]"
  Demux/1 -> KT/1  "Corriente [A]"
  Acond/1 -> Scope1/1, Wm_s [V]/1
  Sensor Encoder/1 -> Acond/1
  Demux/2 -> Sensor Encoder/1  "x2"
  Wdot/1 -> Planta Motor/2(w_dot)  "Acc Ang [rad/s2]"
  Vin/1 -> Scope/1, Planta Motor/1(U)

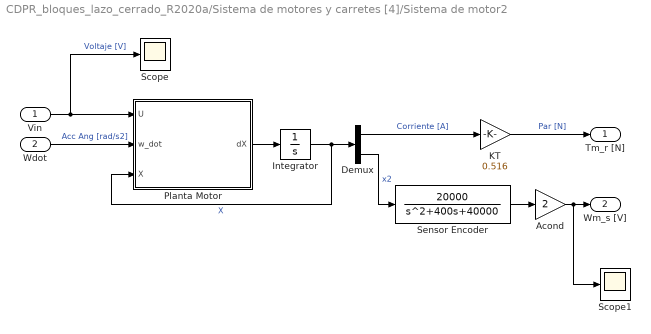
== system CDPR_bloques_lazo_cerrado_R2020a/Sistema de motores y carretes [4]/Sistema de motor2 ==
  Vin : Inport
  Wdot : Inport  Port=2
  Acond : Gain  Gain=2
  Demux : Demux  Outputs=2
  Integrator : Integrator  InitialCondition=[0 0]
  KT : Gain  Gain=0.516
  Planta Motor : MATLAB Function  TreatAsAtomicUnit=on
  Scope : Scope
  Scope1 : Scope
  Sensor Encoder : TransferFcn  Numerator=[20000]  Denominator=[1 400 40000]
  Tm_r [N] : Outport
  Wm_s [V] : Outport  Port=2
  wires:
  Planta Motor/1(dX) -> Integrator/1
  Integrator/1 -> Planta Motor/3(X), Demux/1  "X"
  KT/1 -> Tm_r [N]/1  "Par [N]"
  Demux/1 -> KT/1  "Corriente [A]"
  Wdot/1 -> Planta Motor/2(w_dot)  "Acc Ang [rad/s2]"
  Vin/1 -> Scope/1, Planta Motor/1(U)  "Voltaje [V]"
  Acond/1 -> Scope1/1, Wm_s [V]/1
  Sensor Encoder/1 -> Acond/1
  Demux/2 -> Sensor Encoder/1  "x2"

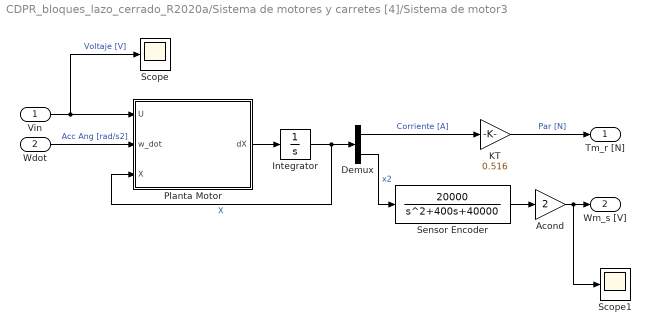
== system CDPR_bloques_lazo_cerrado_R2020a/Sistema de motores y carretes [4]/Sistema de motor3 ==
  Vin : Inport
  Wdot : Inport  Port=2
  Acond : Gain  Gain=2
  Demux : Demux  Outputs=2
  Integrator : Integrator  InitialCondition=[0 0]
  KT : Gain  Gain=0.516
  Planta Motor : MATLAB Function  TreatAsAtomicUnit=on
  Scope : Scope
  Scope1 : Scope
  Sensor Encoder : TransferFcn  Numerator=[20000]  Denominator=[1 400 40000]
  Tm_r [N] : Outport
  Wm_s [V] : Outport  Port=2
  wires:
  Planta Motor/1(dX) -> Integrator/1
  Integrator/1 -> Planta Motor/3(X), Demux/1  "X"
  KT/1 -> Tm_r [N]/1  "Par [N]"
  Demux/1 -> KT/1  "Corriente [A]"
  Wdot/1 -> Planta Motor/2(w_dot)  "Acc Ang [rad/s2]"
  Vin/1 -> Scope/1, Planta Motor/1(U)  "Voltaje [V]"
  Acond/1 -> Scope1/1, Wm_s [V]/1
  Sensor Encoder/1 -> Acond/1
  Demux/2 -> Sensor Encoder/1  "x2"

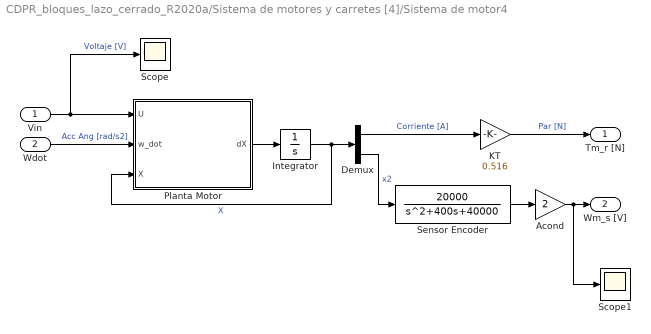
== system CDPR_bloques_lazo_cerrado_R2020a/Sistema de motores y carretes [4]/Sistema de motor4 ==
  Vin : Inport
  Wdot : Inport  Port=2
  Acond : Gain  Gain=2
  Demux : Demux  Outputs=2
  Integrator : Integrator  InitialCondition=[0 0]
  KT : Gain  Gain=0.516
  Planta Motor : MATLAB Function  TreatAsAtomicUnit=on
  Scope : Scope
  Scope1 : Scope
  Sensor Encoder : TransferFcn  Numerator=[20000]  Denominator=[1 400 40000]
  Tm_r [N] : Outport
  Wm_s [V] : Outport  Port=2
  wires:
  Planta Motor/1(dX) -> Integrator/1
  Integrator/1 -> Planta Motor/3(X), Demux/1  "X"
  KT/1 -> Tm_r [N]/1  "Par [N]"
  Demux/1 -> KT/1  "Corriente [A]"
  Wdot/1 -> Planta Motor/2(w_dot)  "Acc Ang [rad/s2]"
  Vin/1 -> Scope/1, Planta Motor/1(U)  "Voltaje [V]"
  Acond/1 -> Scope1/1, Wm_s [V]/1
  Sensor Encoder/1 -> Acond/1
  Demux/2 -> Sensor Encoder/1  "x2"

== matlab function CDPR_bloques_lazo_cerrado_R2020a/Sistema de motores y carretes [4]/Sistema de motor4/Planta Motor ==
  data: U input; w_dot input; dX output; X input
function dX  = MotorCD(U, w_dot, X)
%Parametros del sistema

Kb = 1.25;
Kt = 0.516;
Jm = 0.0221;
Bm = 0.002953;
Ra = 2.581;
La = 0.0281;

a11 = -Ra/La;
a12 = -Kb/La;
a21 =  Kt/Jm;
a22 = -Bm/Jm;
b11 = 1/La;
b22 = 0;
f11 = 0;
f22 = -1/Jm;
 
A = [a11 a12; a21 a22]; 
B = [b11; b22];

F = [f11; f22];
TL = -Kt * X(1) + Jm * w_dot + Bm * X(2) ;
 
dX = A*X + B*U + F*TL;
end

== matlab function CDPR_bloques_lazo_cerrado_R2020a/Controladores y observadores Motores DC [4] /Controlador y Observador Motor CD2/MATLAB Function ==
  settings: updateMethod=CONTINUOUS
  data: ref input; X input; U output
function U  = Controlador(ref, X)
Kb = 1.25;
Kt = 0.516;
Jm = 0.0221;
Bm = 0.002953;
Ra = 2.581;
La = 0.0281;

a11 = -Ra/La;
a12 = -Kb/La;
a21 =  Kt/Jm;
a22 = -Bm/Jm;
b11 = 1/La;
b22 = 0;
 
A = [a11 a12; a21 a22]; 
B = [b11; b22];
C = [Kt 0];
Pd = [-4 -4];
%Controlador
Mc = [B A*B];
H = (A-Pd(1)*eye(2))*(A-Pd(2)*eye(2));
K = -[0 1] * inv(Mc) * H;
F = 1/(C*inv(-A-B*K) * B);

U = K*X + F*ref;
end

== matlab function CDPR_bloques_lazo_cerrado_R2020a/Controladores y observadores Motores DC [4] /Controlador y Observador Motor CD2/MATLAB Function2 ==
  data: U input; X input; Y_err input; dX_hat output
function dX_hat = Observador(U, X, Y_err)
Kb = 1.25;
Kt = 0.516;
Jm = 0.0221;
Bm = 0.002953;
Ra = 2.581;
La = 0.0281;

a11 = -Ra/La;
a12 = -Kb/La;
a21 =  Kt/Jm;
a22 = -Bm/Jm;
b11 = 1/La;
b22 = 0;
 
A = [a11 a12; a21 a22]; 
B = [b11; b22];
C = [0 1];

Pdo = [-80 -80];

Mo1 = [C ;
      C*A];
Ho = (A-Pdo(1)*eye(2))*(A-Pdo(2)*eye(2));
L = -Ho * inv(Mo1) * [0 1].';
%Espacio de estados
dX_hat = A*X + B*U - L*Y_err;
end

== matlab function CDPR_bloques_lazo_cerrado_R2020a/Controladores y observadores Motores DC [4] /Controlador y Observador Motor CD3/MATLAB Function ==
  settings: updateMethod=CONTINUOUS
  data: ref input; X input; U output
function U  = Controlador(ref, X)
Kb = 1.25;
Kt = 0.516;
Jm = 0.0221;
Bm = 0.002953;
Ra = 2.581;
La = 0.0281;

a11 = -Ra/La;
a12 = -Kb/La;
a21 =  Kt/Jm;
a22 = -Bm/Jm;
b11 = 1/La;
b22 = 0;
 
A = [a11 a12; a21 a22]; 
B = [b11; b22];
C = [Kt 0];
Pd = [-4 -4];
%Controlador
Mc = [B A*B];
H = (A-Pd(1)*eye(2))*(A-Pd(2)*eye(2));
K = -[0 1] * inv(Mc) * H;
F = 1/(C*inv(-A-B*K) * B);

U = K*X + F*ref;
end

== matlab function CDPR_bloques_lazo_cerrado_R2020a/Controladores y observadores Motores DC [4] /Controlador y Observador Motor CD3/MATLAB Function2 ==
  data: U input; X input; Y_err input; dX_hat output
function dX_hat = Observador(U, X, Y_err)
Kb = 1.25;
Kt = 0.516;
Jm = 0.0221;
Bm = 0.002953;
Ra = 2.581;
La = 0.0281;

a11 = -Ra/La;
a12 = -Kb/La;
a21 =  Kt/Jm;
a22 = -Bm/Jm;
b11 = 1/La;
b22 = 0;
 
A = [a11 a12; a21 a22]; 
B = [b11; b22];
C = [0 1];

Pdo = [-80 -80];

Mo1 = [C ;
      C*A];
Ho = (A-Pdo(1)*eye(2))*(A-Pdo(2)*eye(2));
L = -Ho * inv(Mo1) * [0 1].';
%Espacio de estados
dX_hat = A*X + B*U - L*Y_err;
end

== matlab function CDPR_bloques_lazo_cerrado_R2020a/Controladores y observadores Motores DC [4] /Controlador y Observador Motor CD4/MATLAB Function ==
  settings: updateMethod=CONTINUOUS
  data: ref input; X input; U output
function U  = Controlador(ref, X)
Kb = 1.25;
Kt = 0.516;
Jm = 0.0221;
Bm = 0.002953;
Ra = 2.581;
La = 0.0281;

a11 = -Ra/La;
a12 = -Kb/La;
a21 =  Kt/Jm;
a22 = -Bm/Jm;
b11 = 1/La;
b22 = 0;
 
A = [a11 a12; a21 a22]; 
B = [b11; b22];
C = [Kt 0];
Pd = [-4 -4];
%Controlador
Mc = [B A*B];
H = (A-Pd(1)*eye(2))*(A-Pd(2)*eye(2));
K = -[0 1] * inv(Mc) * H;
F = 1/(C*inv(-A-B*K) * B);

U = K*X + F*ref;
end

== matlab function CDPR_bloques_lazo_cerrado_R2020a/Controladores y observadores Motores DC [4] /Controlador y Observador Motor CD4/MATLAB Function2 ==
  data: U input; X input; Y_err input; dX_hat output
function dX_hat = Observador(U, X, Y_err)
Kb = 1.25;
Kt = 0.516;
Jm = 0.0221;
Bm = 0.002953;
Ra = 2.581;
La = 0.0281;

a11 = -Ra/La;
a12 = -Kb/La;
a21 =  Kt/Jm;
a22 = -Bm/Jm;
b11 = 1/La;
b22 = 0;
 
A = [a11 a12; a21 a22]; 
B = [b11; b22];
C = [0 1];

Pdo = [-80 -80];

Mo1 = [C ;
      C*A];
Ho = (A-Pdo(1)*eye(2))*(A-Pdo(2)*eye(2));
L = -Ho * inv(Mo1) * [0 1].';
%Espacio de estados
dX_hat = A*X + B*U - L*Y_err;
end

== matlab function CDPR_bloques_lazo_cerrado_R2020a/Planta End Effector/MATLAB Function1 ==
  data: JL input; JL_T output
function JL_T = fcn(JL)

JL_T=JL';

== matlab function CDPR_bloques_lazo_cerrado_R2020a/Controlador Planta/MATLAB Function6 ==
  settings: updateMethod=CONTINUOUS
  data: Yref output; clock input; dYref output; ddYref output
function [Yref, dYref, ddYref]  = Ref(clock)
t = clock; 
Yref = [15*sin(t);15*cos(t);15];
dYref = [15*cos(t);-15*sin(t);0];
ddYref = [-15*sin(t);15*cos(t);0];
end

== matlab function CDPR_bloques_lazo_cerrado_R2020a/Jacobiano/MATLAB Function ==
  data: L input; Q output
function Q = Cable_length(L)
Q = zeros(1,4);
    for i = 1 : 4
        qi = (L(:,i).' * L(:,i)) ^(1/2) ;
        Q(:,i) = qi;
    end
end

== matlab function CDPR_bloques_lazo_cerrado_R2020a/Jacobiano/MATLAB Function1 ==
  data: L input; Q input; JT output
function JT   = Jacobian(L,Q)
JT = zeros(3,4);
    for i = 1 : 4
        Ji = (L(:,i)/Q(:,i)) ;
        JT(:,i) = Ji;
    end
end

== matlab function CDPR_bloques_lazo_cerrado_R2020a/Planta End Effector/MATLAB Function ==
  data: U input; dX output; X input; p_acc output; Jt input; p_vel output
function [dX, p_acc, p_vel]  = PlantaEndEffector(U, X, Jt)
%MATRICES
M=70;
Fext=[0;0;-9.81*M];
ZeroI33 = 0 * eye(3);
a11 = ZeroI33;
a12 = ZeroI33;
a21 = eye(3);
a22 = ZeroI33;
b11 = zeros(3,4);
b21 = (-1/M) * Jt;
c11 = eye(3);
c12 = ZeroI33;
d12 = 1/M*Fext;

f = [0;0;0; d12];

A = [a11 a21; a12 a22];
B = [b11; b21];
C = [c11 c12];
 
dX = A*X + B*U + f ;
p_vel = dX(1:3);
p_acc = dX(4:6);
end

== matlab function CDPR_bloques_lazo_cerrado_R2020a/Controladores y observadores Motores DC [4] /Controlador y Observador Motor CD1/MATLAB Function ==
  settings: updateMethod=CONTINUOUS
  data: ref input; X input; U output
function U  = Controlador(ref, X)
Kb = 1.25;
Kt = 0.516;
Jm = 0.0221;
Bm = 0.002953;
Ra = 2.581;
La = 0.0281;

a11 = -Ra/La;
a12 = -Kb/La;
a21 =  Kt/Jm;
a22 = -Bm/Jm;
b11 = 1/La;
b22 = 0;
 
A = [a11 a12; a21 a22]; 
B = [b11; b22];
C = [Kt 0];
Pd = [-4 -4];
%Controlador
Mc = [B A*B];
H = (A-Pd(1)*eye(2))*(A-Pd(2)*eye(2));
K = -[0 1] * inv(Mc) * H;
F = 1/(C*inv(-A-B*K) * B);

U = K*X + F*ref;
end

== matlab function CDPR_bloques_lazo_cerrado_R2020a/Controladores y observadores Motores DC [4] /Controlador y Observador Motor CD1/MATLAB Function2 ==
  data: U input; X input; Y_err input; dX_hat output
function dX_hat = Observador(U, X, Y_err)
Kb = 1.25;
Kt = 0.516;
Jm = 0.0221;
Bm = 0.002953;
Ra = 2.581;
La = 0.0281;

a11 = -Ra/La;
a12 = -Kb/La;
a21 =  Kt/Jm;
a22 = -Bm/Jm;
b11 = 1/La;
b22 = 0;
 
A = [a11 a12; a21 a22]; 
B = [b11; b22];
C = [0 1];

Pdo = [-80 -80];

Mo1 = [C ;
      C*A];
Ho = (A-Pdo(1)*eye(2))*(A-Pdo(2)*eye(2));
L = -Ho * inv(Mo1) * [0 1].';
%Espacio de estados
dX_hat = A*X + B*U - L*Y_err;
end

== matlab function CDPR_bloques_lazo_cerrado_R2020a/Sistema de motores y carretes [4]/Sistema de motor2/Planta Motor ==
  data: U input; w_dot input; dX output; X input
function dX  = MotorCD(U, w_dot, X)
%Parametros del sistema

Kb = 1.25;
Kt = 0.516;
Jm = 0.0221;
Bm = 0.002953;
Ra = 2.581;
La = 0.0281;

a11 = -Ra/La;
a12 = -Kb/La;
a21 =  Kt/Jm;
a22 = -Bm/Jm;
b11 = 1/La;
b22 = 0;
f11 = 0;
f22 = -1/Jm;
 
A = [a11 a12; a21 a22]; 
B = [b11; b22];

F = [f11; f22];
TL = -Kt * X(1) + Jm * w_dot + Bm * X(2) ;
 
dX = A*X + B*U + F*TL;
end

== matlab function CDPR_bloques_lazo_cerrado_R2020a/Controlador Planta/MATLAB Function7 ==
  settings: updateMethod=CONTINUOUS
  data: Yref input; dYref input; ddYref input; Jt input; X input; U output; Err output; Xref output
function [U, Err, Xref]  = Controlador(Yref, dYref, ddYref, Jt, X)
% Ubicación de los polos para que el error converja a cero
k1 = -20;            % Pd bloque 1
k2 = -20;            % Pd bloque 2
m = 70;            % valor de la masa
b2 = (-1/m) * Jt;   % valor del B(2);
P = [ 0; 0; -9.81];

% Expresion de los estados; 
x1 = X(1:3);
x2 = X(4:6);

% Ecuaciones de bloques, derivadas de los estados. 
dx1 = x2; 
%dx2 = b2*u + fext;

% Ecuaciones del bloque 1
e1 = Yref - x1;                                                     % 5.4
de1 =  k1 * e1;                                                     % 5.5a
x2ref = dYref  - de1;                                               % 5.6b

% Dinamica de x3ref
dx2ref = ddYref - k1*dYref + k1*dx1;                                % 5.8

% Ecuaciones del bloque 2
e2 = x2ref - x2;                                                    % 5.9
de2 = k2*e2;                                                        % 5.10a

% Salidas del bloque, Ley de control, error y estados de referencia.
U = (pinv(b2))*(dx2ref - de2 - P);                         % 5.16b

Err = [e1; e2];
Xref = x2ref;
end

== matlab function CDPR_bloques_lazo_cerrado_R2020a/Sistema de motores y carretes [4]/Sistema de motor3/Planta Motor ==
  data: U input; w_dot input; dX output; X input
function dX  = MotorCD(U, w_dot, X)
%Parametros del sistema

Kb = 1.25;
Kt = 0.516;
Jm = 0.0221;
Bm = 0.002953;
Ra = 2.581;
La = 0.0281;

a11 = -Ra/La;
a12 = -Kb/La;
a21 =  Kt/Jm;
a22 = -Bm/Jm;
b11 = 1/La;
b22 = 0;
f11 = 0;
f22 = -1/Jm;
 
A = [a11 a12; a21 a22]; 
B = [b11; b22];

F = [f11; f22];
TL = -Kt * X(1) + Jm * w_dot + Bm * X(2) ;
 
dX = A*X + B*U + F*TL;
end

== matlab function CDPR_bloques_lazo_cerrado_R2020a/Sistema de motores y carretes [4]/Sistema de motor1/Planta Motor ==
  data: U input; w_dot input; dX output; X input
function dX  = MotorCD(U, w_dot, X)
%Parametros del sistema

Kb = 1.25;
Kt = 0.516;
Jm = 0.0221;
Bm = 0.002953;
Ra = 2.581;
La = 0.0281;

a11 = -Ra/La;
a12 = -Kb/La;
a21 =  Kt/Jm;
a22 = -Bm/Jm;
b11 = 1/La;
b22 = 0;
f11 = 0;
f22 = -1/Jm;
 
A = [a11 a12; a21 a22]; 
B = [b11; b22];

F = [f11; f22];
TL = -Kt * X(1) + Jm * w_dot + Bm * X(2) ;
 
dX = A*X + B*U + F*TL;
end

== matlab function CDPR_bloques_lazo_cerrado_R2020a/Planta End Effector/MATLAB Function2 ==
  data: J input; JdotQdot output; p_vel input
function JdotQdot = fcn(J, p_vel)
G = gradient(J);
JdotQdot = G * p_vel;
